simulink library "Lib_PFSys_Inverter_TMATS"  (R2018a)
settings: Solver=ode45  StartTime=0.0  StopTime=10.0  RelTol=1e-3  EnableMultiTasking=on
libraries: Lib_PF_BusLoadDC_TMATS x1, Lib_PF_ActiveConvEffDC2DC_TMATS x1
Description:
  | Thomas Modules
settings Model: Creator=jwchapm2  LastModifiedBy=mebell
settings DataIOCC: LimitDataPoints=on  SaveFormat=Array
settings OptimizationCC: ExpressionDepthLimit=2147483647  LifeSpan=inf
settings DebuggingCC: UnderspecifiedInitializationDetection=Classic  MergeDetectMultiDrivingBlocksExec=none  SolverPrmCheckMsg=warning  StateNameClashWarn=warning  SFUnexpectedBacktrackingDiag=warning  SFNoUnconditionalDefaultTransitionDiag=warning  SFExecutionAtInitializationDiag=none
settings HardwareCC: ProdBitPerPointer=32  ProdBitPerSizeT=32  ProdBitPerPtrDiffT=32  ProdLargestAtomicFloat=None  ProdIntDivRoundTo=Undefined  ProdEndianess=Unspecified  ProdWordSize=32  ProdHWDeviceType=32-bit Generic
settings ModelReferenceCC: PropagateSignalLabelsOutOfModel=off
settings CodeAppCC: StateflowObjectComments=on
settings GRTTargetCC: TargetLangStandard=C89/C90 (ANSI)  GeneratePreprocessorConditionals=Disable all
settings ConfigComp: CovMetricSettings=dw  CovHtmlReporting=on  CovSaveCumulativeToWorkspaceVar=on  CovSaveSingleToWorkspaceVar=on  CovExternalEMLEnable=off

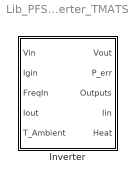
== system Lib_PFSys_Inverter_TMATS ==
  "Inverter " : Subsystem  mask(Inverter){Hz_to_V_M=22, X_C_VoltageVec_M=[0.0 0.1 1.0], Y_C_CurrentVec_M=[0.0 0.1 1.0], T_C_EffArray_M=[0.5 0.5 0.5; 0.5 1.0 1.0; 0.5 1.0 1.0], Pdis_M=1}
      mask prompts: Hz_to_V_M "Hz_to_V_M - Voltage/Flux Constant"; X_C_VoltageVec_M "X_C_VoltageVec_M - Efficiency Table Voltage Vector (X-axis)(nx1), V"; Y_C_CurrentVec_M "Y_C_CurrentVec_M - Efficiency Table Current Vector (Y-axis)(mx1), A"; T_C_EffArray_M "T_C_EffArray_M - Efficiency Table Values (Eff = f(i, V)(nxm)"; Pdis_M "Pdis_M - Constant Power Leaked/Dissipated, W"
      mask help:
      | This block represents a DC-to-AC inverter (for motor control). The block
      | produces an output voltage that scales with input frequency accoring to
      | the flux constant, Hz_to_V_M. The load is assumed to have no inductance,
      | and so we are assumed to operate with unity power factor. Converter
      | efficiency is specified via a lookup table that is a function of output
      | voltage and output current.

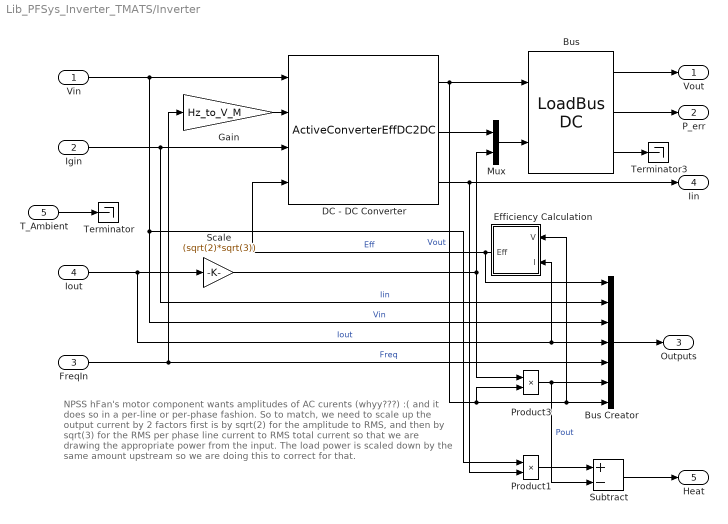
== system Lib_PFSys_Inverter_TMATS/Inverter  ==
  note: NPSS hFan's motor component wants amplitudes of AC curents (whyy???) :(
      | and it does so in a per-line or per-phase fashion.
      | So to match, we need to scale up the output current by 2 factors
      | first is by sqrt(2) for the amplitude to RMS,
      | and then by sqrt(3) for the RMS per phase line current to RMS total current
      | so that we are drawing the appropriate power from the input.
      | The load power is scaled down by the same amount upstream
      | so we are doing this to correct for that.
  Vin : Inport
  Igin : Inport  Port=2
  FreqIn : Inport  Port=3
  Iout : Inport  Port=4
  "T_Ambient " : Inport  Port=5
  Bus : Lib_PF_BusLoadDC_TMATS/LoadBus DC  PeInEN_M=off  P_M=-Pdis_M  BlkNm_M=double(gcb)
  Bus Creator : BusCreator  Inputs=7
  DC - DC Converter : Lib_PF_ActiveConvEffDC2DC_TMATS/ActiveConverterEffDC2DC  EffInEN_M=on  Eff_M=98  BlkNm_M=double(gcb)
  Efficiency Calculation : Subsystem
  Gain : Gain  Gain=Hz_to_V_M
  Mux : Mux  Inputs=2
  Product1 : Product
  Product3 : Product
  Scale : Gain  Gain=(sqrt(2)*sqrt(3))
  Subtract : Sum  Inputs=+-
  Terminator : Terminator
  Terminator3 : Terminator
  Vout : Outport
  P_err : Outport  Port=2
  Outputs : Outport  Port=3
  Iin : Outport  Port=4
  "Heat " : Outport  Port=5
  wires:
  DC - DC Converter/2 -> Mux/1
  Scale/1 -> Mux/2, Product3/1
  Product3/1 -> Bus Creator/6, Subtract/2  "Pout"
  Bus Creator/1 -> Outputs/1
  FreqIn/1 -> Bus Creator/5, Gain/1  "Freq"
  Efficiency Calculation/1(Eff) -> DC - DC Converter/4, Bus Creator/1  "Eff"
  Mux/1 -> Bus/2
  Igin/1 -> DC - DC Converter/3, Bus Creator/2  "Iin"
  Bus/3 -> Terminator3/1
  DC - DC Converter/1 -> Product3/2, Bus Creator/7, Efficiency Calculation/1(V), Bus/1  "Vout"
  Vin/1 -> Bus Creator/3, Product1/1, DC - DC Converter/1  "Vin"
  Gain/1 -> DC - DC Converter/2
  Iout/1 -> Bus Creator/4, Efficiency Calculation/2(I), Scale/1  "Iout"
  DC - DC Converter/3 -> Product1/2, Iin/1
  Bus/2 -> P_err/1
  Bus/1 -> Vout/1
  Product1/1 -> Subtract/1
  Subtract/1 -> "Heat "/1
  "T_Ambient "/1 -> Terminator/1

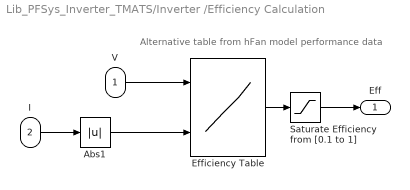
== system Lib_PFSys_Inverter_TMATS/Inverter /Efficiency Calculation ==
  note: Alternative table from hFan model performance data
  V : Inport
  I : Inport  Port=2
  Abs1 : Abs
  Efficiency Table : Lookup_n-D  BreakpointsForDimension1=X_C_VoltageVec_M  BreakpointsForDimension2=Y_C_CurrentVec_M  Table=T_C_EffArray_M  ExtrapMethod=Clip  InternalRulePriority=Speed  RndMeth=Simplest  InputSameDT=on
  Saturate Efficiency from [0.1 to 1] : Saturate  UpperLimit=1  LowerLimit=0.1
  Eff : Outport
  wires:
  Abs1/1 -> Efficiency Table/2
  Saturate Efficiency from [0.1 to 1]/1 -> Eff/1
  Efficiency Table/1 -> Saturate Efficiency from [0.1 to 1]/1
  I/1 -> Abs1/1
  V/1 -> Efficiency Table/1
